simulink model "StepXYQXFzsp"  (Simulink 8.3)
settings: Solver=ode45  StartTime=0.0  StopTime=6000  RelTol=1e-3
values from neighbouring files (symbols this model uses):
  kd = kp*pi/(4*wr)    [ZieglerDm4_29.m]    (also in Zieglerm4_27.m; example4_15.m = 0.01; example4_16.m = 0.006)
  ki = kp*wr/pi    [ZieglerDm4_29.m]    (also in Zieglerm4_27.m; example4_15.m = 1; example4_16.m = 0.01)
  kp = 0.6*kr    [ZieglerDm4_29.m]    (also in Zieglerm4_27.m; example4_15.m = 1.5; example4_16.m = 1.9)
libraries: simulink_need_slupdate x2
settings Model: Creator=sony  LastModifiedBy=sony  ExtModeTrigMode=oneshot  ExtModeArmWhenConnect=off
settings DataIOCC: LimitDataPoints=off  SignalLoggingName=sigsOut
settings OptimizationCC: BooleanDataType=off
settings DebuggingCC: SaveWithParameterizedLinksMsg=none  SignalResolutionControl=TryResolveAllWithWarning  SolverPrmCheckMsg=none  MultiTaskDSMMsg=warning  MultiTaskCondExecSysMsg=none  StateNameClashWarn=none  StrictBusMsg=None
settings HardwareCC: TargetUnknown=on
settings RTWCC: IncludeERTFirstTime=on

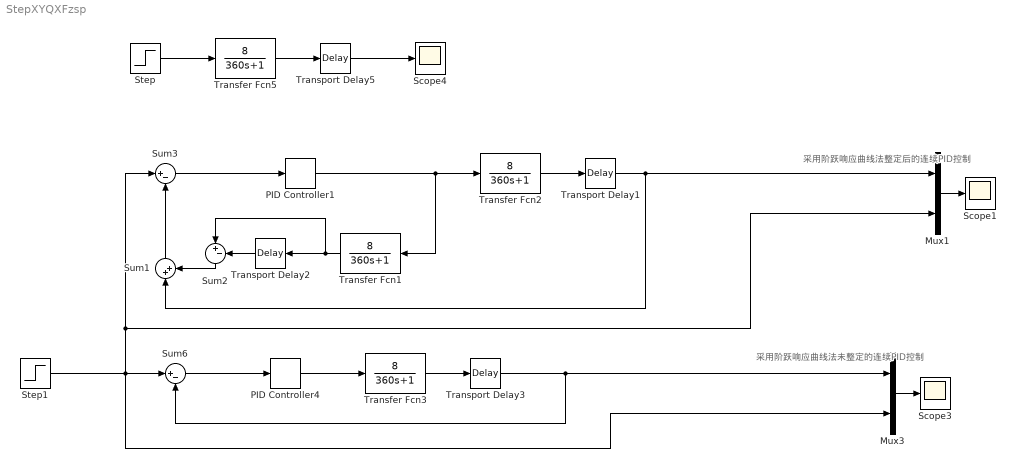
== system StepXYQXFzsp ==
  note: 采用阶跃响应曲线法整定后的连续PID控制
  note: 采用阶跃响应曲线法未整定的连续PID控制
  Mux1 : Mux  Inputs=2
  Mux3 : Mux  Inputs=2
  PID Controller1 : simulink_need_slupdate/PID Controller  P=1.2  I=0.0023  D=18
  PID Controller4 : simulink_need_slupdate/PID Controller  P=kp  I=ki  D=kd
  Scope1 : Scope
      settings: YMin=-3.5  YMax=1  MaxDataPoints=500000
  Scope3 : Scope
      settings: YMin=0  YMax=110  SaveName=ScopeData3  MaxDataPoints=500000
  Scope4 : Scope
      settings: YMin=0  YMax=80  SaveName=S1  MaxDataPoints=500000
  Step : Step  Time=0  SampleTime=0
  Step1 : Step  Time=0  After=50  SampleTime=0
  Sum1 : Sum  Inputs=|++  SaturateOnIntegerOverflow=on
  Sum2 : Sum  Inputs=|+-  SaturateOnIntegerOverflow=on
  Sum3 : Sum  Inputs=|+-  SaturateOnIntegerOverflow=on
  Sum6 : Sum  Inputs=|+-  SaturateOnIntegerOverflow=on
  Transfer Fcn{1..3,5} (4 alike) : TransferFcn  Numerator=[8]  Denominator=[360 1]
  Transport Delay{1..3,5} (4 alike) : TransportDelay  DelayTime=180
  wires:
  Transfer Fcn5/1 -> Transport Delay5/1
  Step1/1 -> Mux1/2, Sum3/1, Mux3/2, Sum6/1
  Transport Delay3/1 -> Sum6/2, Mux3/1
  PID Controller4/1 -> Transfer Fcn3/1
  Sum6/1 -> PID Controller4/1
  Mux3/1 -> Scope3/1
  Transport Delay1/1 -> Sum1/1, Mux1/1
  PID Controller1/1 -> Transfer Fcn2/1, Transfer Fcn1/1
  Sum3/1 -> PID Controller1/1
  Transfer Fcn1/1 -> Transport Delay2/1, Sum2/1
  Transport Delay2/1 -> Sum2/2
  Sum1/1 -> Sum3/2
  Mux1/1 -> Scope1/1
  Sum2/1 -> Sum1/2
  Step/1 -> Transfer Fcn5/1
  Transport Delay5/1 -> Scope4/1
  Transfer Fcn2/1 -> Transport Delay1/1
  Transfer Fcn3/1 -> Transport Delay3/1
